simulink model "flanger_short"  (R2018a)
settings: Solver=FixedStepDiscrete  StartTime=0.0  StopTime=30.0  RelTol=1e-3
libraries: dspvision x2, dspsrcs4 x1, dspsigops x1
settings Model: DataTypeOverride=Off  Creator=Lu  LastModifiedBy=Lu
settings DataIOCC: SaveOutput=off  SaveTime=off
settings OptimizationCC: BlockReduction=off  ConditionallyExecuteInputs=off  DefaultParameterBehavior=Inlined
settings DebuggingCC: AlgebraicLoopMsg=error  SingleTaskRateTransMsg=error
settings HardwareCC: ProdBitPerPointer=32  ProdBitPerSizeT=32  ProdBitPerPtrDiffT=32  ProdLargestAtomicFloat=None  ProdIntDivRoundTo=Undefined  ProdEndianess=Unspecified  ProdWordSize=32  ProdHWDeviceType=ASIC/FPGA->ASIC/FPGA  TargetBitPerPointer=64  TargetBitPerSizeT=64  TargetBitPerPtrDiffT=64  TargetLongLongMode=on  TargetIntDivRoundTo=Zero  TargetEndianess=LittleEndian  TargetWordSize=64  TargetHWDeviceType=Custom Processor->MATLAB Host Computer  ProdEqTarget=off

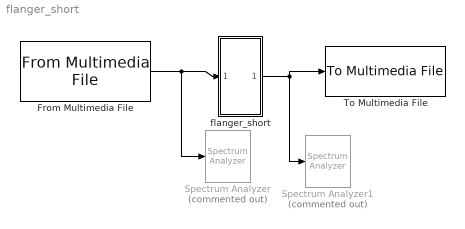
== system flanger_short ==
  From Multimedia File : dspvision/From Multimedia File  inputFilename=C:\Users\lugfe\Documents\GitHub\dsp-fpgay\TP FINAL\audio effects\shook.wav  loop=on  numPlays=1  outputStreams=Audio only  videoDataType=single  audioDataType=int16  inheritSampleTime=on  userDefinedSampleTime=1/30  noAudioOutput=off  isIntensityVideo=off  fourcc=RGB  colorVideoFormat=Separate color signals  outputEOF=off  dataOrg=Column-major  audioFrameSize=1  computeAudioFrameSize=off  outSamplingMode=Sample based
      settings: SourceProductBaseCode=VP
  Spectrum Analyzer : SpectrumAnalyzer  Commented=on
  Spectrum Analyzer1 : SpectrumAnalyzer  Commented=on
  To Multimedia File : dspvision/To Multimedia File  outputFilename=C:\Users\lugfe\Documents\GitHub\dsp-fpgay\TP FINAL\audio effects\flanger_shook.wav  streamSelection=Audio only  videoCompressor=None (uncompressed)  audioCompressor=None (uncompressed)  imagePorts=Separate color signals  fileType=WAV  audioDatatype=Determine from input data type  fourcc=RGB  videoQuality=75  mj2000CompFactor=10
      settings: SourceProductName=Computer Vision System Toolbox  SourceProductBaseCode=VP
  "flanger_short " : Subsystem
  wires:
  From Multimedia File/1 -> Spectrum Analyzer/1, "flanger_short "/1(In2)
  "flanger_short "/1(Out2) -> To Multimedia File/1, Spectrum Analyzer1/1

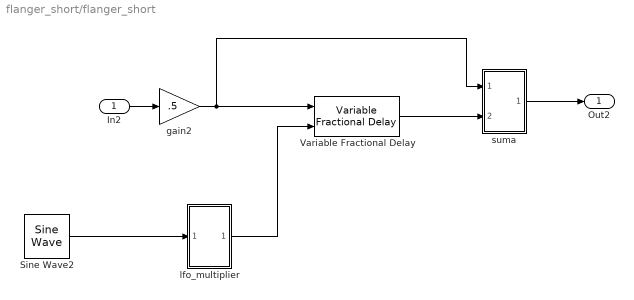
== system flanger_short/flanger_short  ==
  In2 : Inport  OutDataTypeStr=int16  SampleTime=1/44100
  Sine Wave2 : dspsrcs4/Sine Wave  Amplitude=1  Frequency=0.5  Phase=0  SampleMode=Discrete  OutComplex=Real  CompMethod=Table lookup  TableSize=Memory  SampleTime=1/44100  SamplesPerFrame=1  ResetState=Restart at time zero  OutputFrames=off  dataType=Fixed-point  wordLen=16  udDataType=sfix(16)  fracBitsMode=Best precision  numFracBits=14  OutDataTypeStr=fixdt(1,16)  LastOutDataTypeStr=fixdt(1,16)
  Variable Fractional Delay : dspsigops/Variable Fractional Delay  mode=OBSOLETE  modeActive=Linear  dmax=2000  InputProcessing=Columns as channels (frame based)  L=4  FarrowL=4  R=10  alpha=1  ic=0  fallbackFIR=Clip to the minimum value necessary for centered kernel  fallbackFarrow=Clip to the minimum value necessary for centered kernel  noDFT=off  roundingMode=Ceiling  overflowMode=on
      settings: SourceProductName=DSP System Toolbox  SourceProductBaseCode=DS
  gain2 : Gain  Gain=.5  OutDataTypeStr=int16
  "lfo_multiplier " : Subsystem
  "suma " : Subsystem
  Out2 : Outport
  wires:
  gain2/1 -> "suma "/1(In1), Variable Fractional Delay/1
  In2/1 -> gain2/1
  Variable Fractional Delay/1 -> "suma "/2(In2)
  "suma "/1(Out1) -> Out2/1
  Sine Wave2/1 -> "lfo_multiplier "/1(In1)
  "lfo_multiplier "/1(Out1) -> Variable Fractional Delay/2

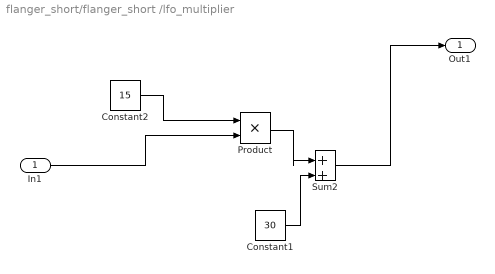
== system flanger_short/flanger_short /lfo_multiplier  ==
  In1 : Inport
  Constant1 : Constant  Value=30  OutDataTypeStr=fixdt(1,16)
  Constant2 : Constant  Value=15  OutDataTypeStr=fixdt(1,16)
  Product : Product  SaturateOnIntegerOverflow=on
  Sum2 : Sum  Inputs=|++  AccumDataTypeStr=fixdt(1,16,0)  RndMeth=Ceiling  SaturateOnIntegerOverflow=on
  Out1 : Outport
  wires:
  Constant1/1 -> Sum2/2
  Product/1 -> Sum2/1
  In1/1 -> Product/2
  Constant2/1 -> Product/1
  Sum2/1 -> Out1/1

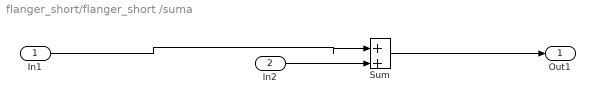
== system flanger_short/flanger_short /suma  ==
  In1 : Inport
  In2 : Inport  Port=2
  Sum : Sum  Inputs=|++  AccumDataTypeStr=int16
  Out1 : Outport
  wires:
  In2/1 -> Sum/2
  Sum/1 -> Out1/1
  In1/1 -> Sum/1
